simulink model "NOLCOLab2Q1"  (R2016b)
settings: Solver=VariableStepAuto  StartTime=0.0  StopTime=10.0  RelTol=1e-3
settings Model: Creator=akshita_jain  LastModifiedBy=akshita_jain

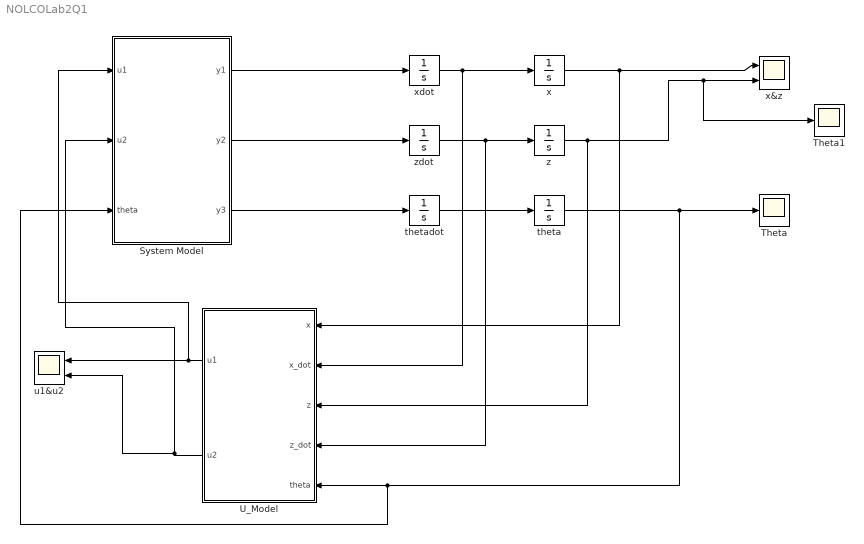
== system NOLCOLab2Q1 ==
  System Model : MATLAB Function  TreatAsAtomicUnit=on
  Theta : Scope
  Theta1 : Scope
  "U_Model " : MATLAB Function  TreatAsAtomicUnit=on
  theta : Integrator  InitialCondition=pi/4
  thetadot : Integrator
  u1&u2 : Scope  NumInputPorts=2
  x : Integrator  InitialCondition=1
  x&z : Scope  NumInputPorts=2
  xdot : Integrator
  z : Integrator  InitialCondition=1
  zdot : Integrator
  wires:
  System Model/1(y1) -> xdot/1
  System Model/2(y2) -> zdot/1
  System Model/3(y3) -> thetadot/1
  xdot/1 -> "U_Model "/2(x_dot), x/1
  zdot/1 -> "U_Model "/4(z_dot), z/1
  thetadot/1 -> theta/1
  z/1 -> "U_Model "/3(z), Theta1/1, x&z/2
  theta/1 -> "U_Model "/5(theta), System Model/3(theta), Theta/1
  "U_Model "/1(u1) -> u1&u2/1, System Model/1(u1)
  "U_Model "/2(u2) -> u1&u2/2, System Model/2(u2)
  x/1 -> "U_Model "/1(x), x&z/1

== matlab function NOLCOLab2Q1/U_Model  ==
  data: x input; u1 output; x_dot input; z input; u2 output; z_dot input; theta input
function [u1,u2]= fcn(x,x_dot,z,z_dot,theta)
eps = 0.001;
% a is decouple matrix 
a = [-sin(theta) eps*cos(theta); cos(theta) eps*sin(theta)];
% b = Gain(output) Matrix + alpha (constants) 
b = [0;1]+[-10*x_dot-25*x; -10*z_dot-25*z];
u = (a^-1)*b; 
u1 = u(1);
u2 = u(2);

end

== matlab function NOLCOLab2Q1/System Model ==
  data: u1 input; y1 output; u2 input; theta input; y2 output; y3 output
function [y1,y2,y3]= fcn(u1,u2,theta)
eps = 0.001;
x_ddot = -sin(theta)*u1 + eps*cos(theta)*u2;
z_ddot = cos(theta)*u1 + eps*sin(theta)*u2 - 1;
theta_ddot = u2;
y1 = x_ddot;
y2 = z_ddot;
y3 = theta_ddot;
